simulink model "hw3_a_RLS_lambda_model_c0"  (R2024b)
settings: Solver=ode4  StartTime=0.0  StopTime=sim_time  FixedStep=sample_time  RelTol=1e-3
values from neighbouring files (symbols this model uses):
  a = -0.8    [hw3_a_rls_v2.m]    (also in hw3_b_rls_v2.m)
  b = 0.5    [hw3_a_rls_v2.m]    (also in hw3_b_rls_v2.m)
  c = -0.5    [hw3_a_rls_v2.m]    (also in hw3_b_rls_v2.m = 0)
  noise_mean = 0    [hw3_a_rls_v2.m]    (also in hw3_b_rls_v2.m)
  noise_seed = round(rand*1e5)    [hw3_a_rls_v2.m]    (also in hw3_b_rls_v2.m)
  noise_variance = 0.5    [hw3_a_rls_v2.m]    (also in hw3_b_rls_v2.m)
  P_0 = eye(3,3) * 100    [hw3_a_rls_v2.m]    (also in hw3_b_rls_v2.m)
  sample_time = 1    [hw3_a_rls_v2.m]    (also in hw3_b_rls_v2.m)
  Theta_0 = [0;0;0]    [hw3_a_rls_v2.m]    (also in hw3_b_rls_v2.m)
libraries: simulink x1
settings Model: Creator=kemal  LastModifiedBy=kemal

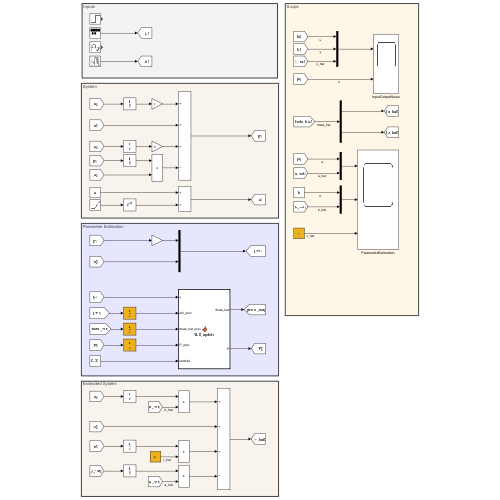
[thumbnail: Simulink's stored preview of the top-level diagram]
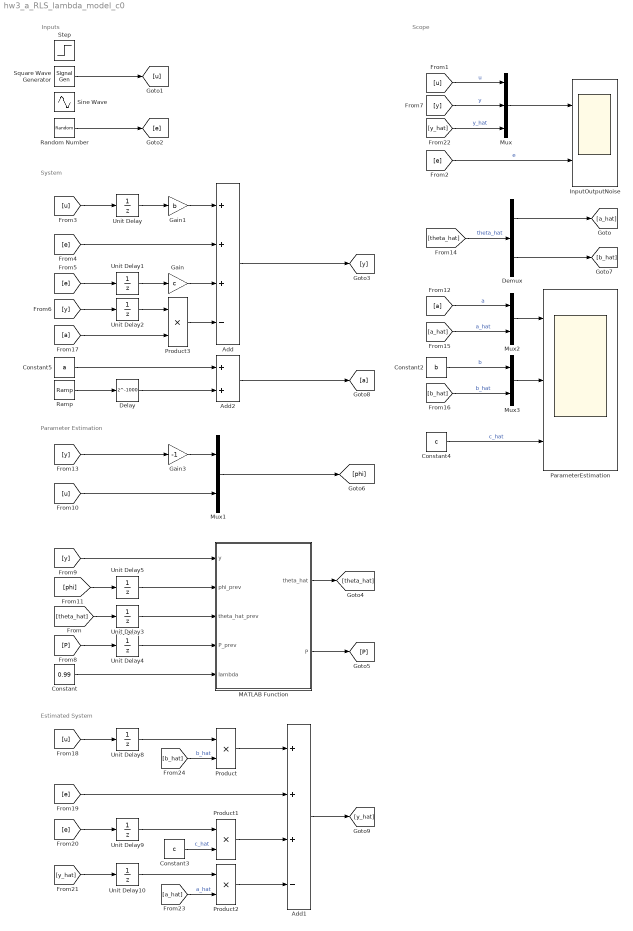
== system hw3_a_RLS_lambda_model_c0 ==
  note: Inputs
  note: System
  note: Scope
  note: Parameter Estimation
  note: Estimated System
  Add : Sum  Inputs=+++-
  Add1 : Sum  Inputs=+++-
  Add2 : Sum
  Constant : Constant  Value=0.99  SampleTime=-1
  Constant2 : Constant  Value=b  SampleTime=sample_time
  Constant3 : Constant  Value=c
  Constant4 : Constant  Value=c
  Constant5 : Constant  Value=a  SampleTime=sample_time
  Delay : Delay  DelayLength=1000  SampleTime=sample_time
  Demux : Demux  Outputs=2
  Gain : Gain  Gain=c
  Gain1 : Gain  Gain=b
  Gain3 : Gain  Gain=-1
  InputOutputNoise : Scope  NumInputPorts=2
  MATLAB Function : MATLAB Function  TreatAsAtomicUnit=on
  Mux : Mux  Inputs=3
  Mux1 : Mux  Inputs=2
  Mux2 : Mux  Inputs=2
  Mux3 : Mux  Inputs=2
  ParameterEstimation : Scope  NumInputPorts=3
  Product{,1..3} (4 alike) : Product
  Ramp : simulink/Sources/Ramp  slope=0.0001*3  start=0  InitialOutput=0
  Random Number : RandomNumber  Mean=noise_mean  Variance=noise_variance  Seed=noise_seed  SampleTime=sample_time
  Sine Wave : Sin  Amplitude=25  Frequency=0.25  SampleTime=sample_time
  Square Wave Generator : SignalGenerator  WaveForm=square  Frequency=1/100
  Step : Step  After=100  SampleTime=0
  Unit Delay{,1..2,5,8..10} (7 alike) : UnitDelay  SampleTime=sample_time  HasFrameUpgradeWarning=on
  Unit Delay3 : UnitDelay  InitialCondition=Theta_0  SampleTime=sample_time  HasFrameUpgradeWarning=on
  Unit Delay4 : UnitDelay  InitialCondition=P_0  SampleTime=sample_time  HasFrameUpgradeWarning=on
  wires:
  [u] -> Unit Delay/1
  [e] -> Unit Delay1/1
  Unit Delay1/1 -> Gain/1
  Unit Delay/1 -> Gain1/1
  Gain/1 -> Add/3
  [e] -> Add/2
  Gain1/1 -> Add/1
  [y] -> Unit Delay2/1
  Unit Delay2/1 -> Product3/1
  Product3/1 -> Add/4
  Add/1 -> [y]
  Square Wave Generator/1 -> [u]
  [u] -> Mux/1  "u"
  [y] -> Mux/2  "y"
  [e] -> InputOutputNoise/2  "e"
  Mux/1 -> InputOutputNoise/1
  Random Number/1 -> [e]
  MATLAB Function/2(P) -> [P]
  MATLAB Function/1(theta_hat) -> [theta_hat]
  [theta_hat] -> Unit Delay3/1
  Unit Delay3/1 -> MATLAB Function/3(theta_hat_prev)
  [P] -> Unit Delay4/1
  Unit Delay4/1 -> MATLAB Function/4(P_prev)
  Constant/1 -> MATLAB Function/5(lambda)
  [y] -> MATLAB Function/1(y)
  [y] -> Gain3/1
  Gain3/1 -> Mux1/1
  Mux1/1 -> [phi]
  [phi] -> Unit Delay5/1
  [theta_hat] -> Demux/1  "theta_hat"
  Mux2/1 -> ParameterEstimation/1
  Mux3/1 -> ParameterEstimation/2
  [a] -> Mux2/1  "a"
  Demux/1 -> [a_hat]
  Demux/2 -> [b_hat]
  Constant2/1 -> Mux3/1  "b"
  [a_hat] -> Mux2/2  "a_hat"
  [b_hat] -> Mux3/2  "b_hat"
  Add1/1 -> [y_hat]
  [y_hat] -> Unit Delay10/1
  Unit Delay8/1 -> Product/1
  [e] -> Unit Delay9/1
  [u] -> Unit Delay8/1
  Product/1 -> Add1/1
  Product1/1 -> Add1/3
  Unit Delay9/1 -> Product1/1
  Product2/1 -> Add1/4
  [b_hat] -> Product/2  "b_hat"
  Constant3/1 -> Product1/2  "c_hat"
  [a_hat] -> Product2/2  "a_hat"
  Unit Delay10/1 -> Product2/1
  [e] -> Add1/2
  [y_hat] -> Mux/3  "y_hat"
  [u] -> Mux1/2
  Unit Delay5/1 -> MATLAB Function/2(phi_prev)
  Constant4/1 -> ParameterEstimation/3  "c_hat"
  Constant5/1 -> Add2/1
  Delay/1 -> Add2/2
  Ramp/1 -> Delay/1
  Add2/1 -> [a]
  [a] -> Product3/2

== matlab function hw3_a_RLS_lambda_model_c0/MATLAB Function ==
  data: y input; theta_hat output; phi_prev input; theta_hat_prev input; P_prev input; lambda input; P output
function [theta_hat, P] = RLS_update(y, phi_prev, theta_hat_prev, P_prev, lambda)
    % Compute innovation
    epsilon = y - phi_prev' * theta_hat_prev;
     
    % Update covariance matrix
    P = (1/lambda) * (P_prev - (P_prev * (phi_prev * phi_prev') * P_prev) / ...
        (lambda + phi_prev' * P_prev * phi_prev));

    % Update parameter estimate
    theta_hat = theta_hat_prev + P * phi_prev * epsilon;
end
